simulink model "dynamics_old_3_12_24"  (R2023b)
settings: Solver=ode45  StartTime=0.0  StopTime=StopTime  FixedStep=.1  RelTol=1e-5
PreLoadFcn:
  | StopTime = 5000; gravity = true; k = 10; b = 100; ktr = 300; btr = 300; d0 = 125; l0 = 515.3882; mu = 398600000000000; mp = 1500; mp_inv = 0.00066667; mtr = 1.6667; mtr_inv = 0.6; NRao0 = [-504.021290494982;4.21156034226775e-10;6878000]; NRbo0 = [504.021290495824;4.21156034226775e-10;6878000]; NRfo0 = [4.21125171823769e-10;4.21125171823769e-10;6877495.9787095]; NRgo0 = [4.2118689662978e-10;4.2118689662978e-10;6878504.0212905]; NRdo0 = [4.21156034226775e-10;-124.968757810126;6878000]; NReo0 = [4.21156034226775e-10;124.968757810969;6878000]; NVao0 = [-7612.67977015526;-3.08624030053628e-16;-5.04021290495356]; NVbo0 = [-7612.67977015526;3.08624030053685e-16;5.04021290495449]; NVfo0 = [-7607.6395572503;2.85240796223787e-29;4.65833571642668e-13]; NVgo0 = [-7617.71998306021;2.85618751654332e-29;4.66450819702776e-13]; NVdo0 = [-7612.67977015526;2.85429773939059e-29;4.66142195672722e-13]; NVeo0 = [-7612.67977015526;2.85429773939059e-29;4.66142195672722e-13];
settings Model: Creator=cyrus  LastModifiedBy=cyrus

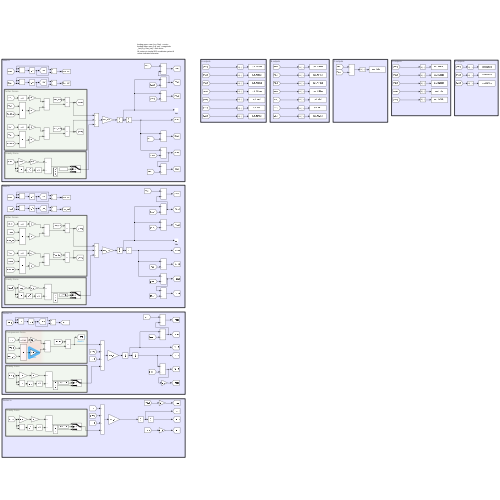
[thumbnail: Simulink's stored preview of the top-level diagram]
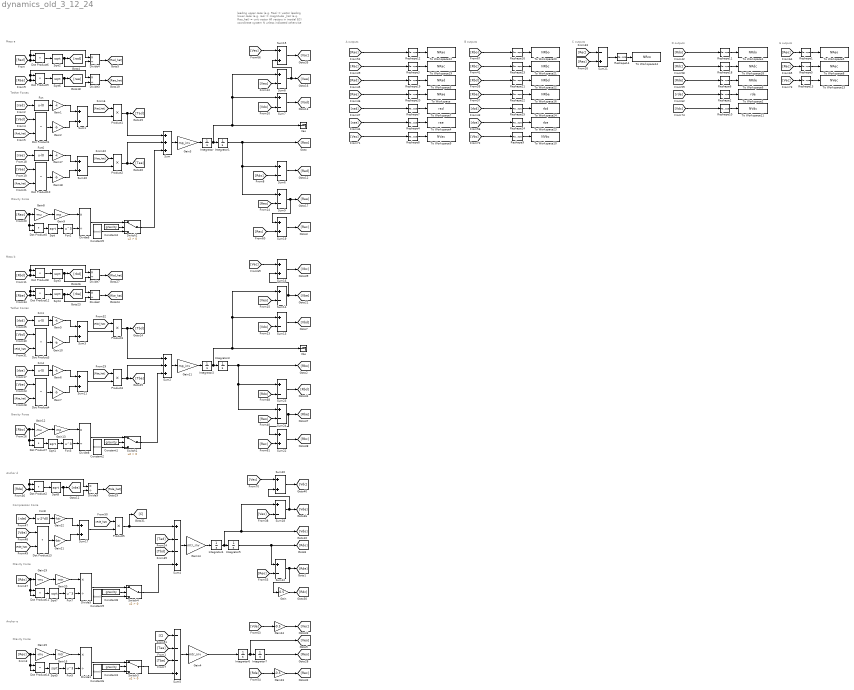
== system dynamics_old_3_12_24 ==
  note: A outputs
  note: Gravity Force
  note: Anchor d
  note: Tether Forces
  note: leading upper case (e.g. Rao) = vector
      | leading lower case (e.g. rao) = magnitude
      | _hat (e.g. Rao_hat) = unit vector
      | All vectors in inertial ECI coordinate system N unless indicated otherwise
  note: Mass a
  note: Gravity Force
  note: Gravity Force
  note: Tether Forces
  note: Mass b
  note: Gravity Force
  note: Anchor e
  note: Compression Force
  note: B outputs
  note: C outputs
  note: D outputs
  note: E outputs
  Constant{1,3..4,8} (4 alike) : Constant  Value=gravity
  Constant{2,5..6,9} (4 alike) : Constant  Value=[0;0;0]  VectorParams1D=off
  Divide{1..9} (9 alike) : Product  Inputs=*/
  Dot Product{1..14} (14 alike) : DotProduct  OutDataTypeStr=Inherit: Inherit via internal rule
  Fcn{,1,4,6} (4 alike) : Fcn  Expr=u-l0
  Fcn{2..3,5,7} (4 alike) : Fcn  Expr=u^3
  Fcn8 : Fcn  Expr=u-2*d0
  Gain : Gain  Gain=0.5
  Gain{1,5..6,17} (4 alike) : Gain  Gain=-k
  Gain{2,7,10,18} (4 alike) : Gain  Gain=-b
  Gain11 : Gain  Gain=mp_inv
  Gain{8,12,15,19} (4 alike) : Gain  Gain=-mu
  Gain13 : Gain  Gain=mp
  Gain14 : Gain  Gain=mtr_inv
  Gain16 : Gain  Gain=mtr
  Gain20 : Gain  Gain=mtr
  Gain21 : Gain  Gain=-btr
  Gain22 : Gain  Gain=-ktr
  Gain23 : Gain  Gain=-0.5
  Gain24 : Gain  Gain=-0.5
  Gain3 : Gain  Gain=mp_inv
  Gain4 : Gain  Gain=mtr_inv
  Gain9 : Gain  Gain=mp
  Integrator : Integrator  InitialCondition=NVao0
  Integrator1 : Integrator  InitialCondition=NRao0
  Integrator2 : Integrator  InitialCondition=NVbo0
  Integrator3 : Integrator  InitialCondition=NRbo0
  Integrator4 : Integrator  InitialCondition=NVdo0
  Integrator5 : Integrator  InitialCondition=NRdo0
  Integrator6 : Integrator  InitialCondition=NVeo0
  Integrator7 : Integrator  InitialCondition=NReo0
  Product{1..5} (5 alike) : Product
  Reshape{1..14,16,18..25} (23 alike) : Reshape
  Sqrt{,1..8} (9 alike) : Sqrt
  Sum : Sum  Inputs=+++
  Sum{1,3,10..11,15..17,19..20,22} (10 alike) : Sum
  Sum{6..9,12..14,18,23..24} (10 alike) : Sum  Inputs=+-
  Sum2 : Sum  Inputs=+++
  Sum21 : Sum  Inputs=-+
  Sum4 : Sum  Inputs=+--+
  Sum5 : Sum  Inputs=---+
  Switch{1..4} (4 alike) : Switch  Criteria=u2 > Threshold  SaturateOnIntegerOverflow=off  InputSameDT=off
  To Workspace : ToWorkspace  VariableName=NRae  SampleTime=-1
  To Workspace1 : ToWorkspace  VariableName=NRdo  SampleTime=-1
      settings: Save2DSignal=2-D array (concatenate along first dimension)
  To Workspace10 : ToWorkspace  VariableName=NVbc  SampleTime=-1
      settings: Save2DSignal=2-D array (concatenate along first dimension)
  To Workspace11 : ToWorkspace  VariableName=NVdc  SampleTime=-1
      settings: Save2DSignal=2-D array (concatenate along first dimension)
  To Workspace12 : ToWorkspace  VariableName=NRao  SampleTime=-1
      settings: Save2DSignal=2-D array (concatenate along first dimension)
  To Workspace13 : ToWorkspace  VariableName=NVec  SampleTime=-1
      settings: Save2DSignal=2-D array (concatenate along first dimension)
  To Workspace14 : ToWorkspace  VariableName=NRco  SampleTime=-1
      settings: Save2DSignal=2-D array (concatenate along first dimension)
  To Workspace16 : ToWorkspace  VariableName=NRbe  SampleTime=-1
  To Workspace18 : ToWorkspace  VariableName=NRdc  SampleTime=-1
      settings: Save2DSignal=2-D array (concatenate along first dimension)
  To Workspace19 : ToWorkspace  VariableName=NRac  SampleTime=-1
      settings: Save2DSignal=2-D array (concatenate along first dimension)
  To Workspace2 : ToWorkspace  VariableName=rde  SampleTime=-1
      settings: Save2DSignal=2-D array (concatenate along first dimension)
  To Workspace20 : ToWorkspace  VariableName=NRbo  SampleTime=-1
      settings: Save2DSignal=2-D array (concatenate along first dimension)
  To Workspace21 : ToWorkspace  VariableName=NRbc  SampleTime=-1
      settings: Save2DSignal=2-D array (concatenate along first dimension)
  To Workspace22 : ToWorkspace  VariableName=NRbd  SampleTime=-1
  To Workspace23 : ToWorkspace  VariableName=rbe  SampleTime=-1
      settings: Save2DSignal=2-D array (concatenate along first dimension)
  To Workspace24 : ToWorkspace  VariableName=rbd  SampleTime=-1
      settings: Save2DSignal=2-D array (concatenate along first dimension)
  To Workspace3 : ToWorkspace  VariableName=NRad  SampleTime=-1
  To Workspace4 : ToWorkspace  VariableName=rae  SampleTime=-1
      settings: Save2DSignal=2-D array (concatenate along first dimension)
  To Workspace5 : ToWorkspace  VariableName=NReo  SampleTime=-1
      settings: Save2DSignal=2-D array (concatenate along first dimension)
  To Workspace6 : ToWorkspace  VariableName=NRde  SampleTime=-1
      settings: Save2DSignal=2-D array (concatenate along first dimension)
  To Workspace7 : ToWorkspace  VariableName=rad  SampleTime=-1
      settings: Save2DSignal=2-D array (concatenate along first dimension)
  To Workspace8 : ToWorkspace  VariableName=NRec  SampleTime=-1
      settings: Save2DSignal=2-D array (concatenate along first dimension)
  To Workspace9 : ToWorkspace  VariableName=NVac  SampleTime=-1
      settings: Save2DSignal=2-D array (concatenate along first dimension)
  Vao : Terminator
  Vbo : Terminator
  wires:
  [Rad] -> Divide4/1, Dot Product6/1, Dot Product6/2
  Dot Product6/1 -> Sqrt2/1
  Sqrt2/1 -> Divide4/2, [rad]
  Divide4/1 -> [Rad_hat]
  [rad] -> Fcn/1
  Fcn/1 -> Gain1/1
  Gain1/1 -> Sum1/1
  [Vad] -> Dot Product1/1
  [Rad_hat] -> Dot Product1/2
  Dot Product1/1 -> Gain2/1
  Gain2/1 -> Sum1/2
  Sum1/1 -> Product1/2
  Sum/1 -> Gain3/1
  Gain3/1 -> Integrator/1
  Integrator/1 -> Integrator1/1, Vao/1, Sum7/1, Sum8/1
  Integrator1/1 -> [Rao], Sum6/1, Sum9/1
  [Rao] -> Dot Product5/2, Dot Product5/1, Gain8/1
  Gain8/1 -> Gain9/1
  Gain9/1 -> Divide6/1
  Fcn2/1 -> Divide6/2
  Sqrt/1 -> Fcn2/1
  Dot Product5/1 -> Sqrt/1
  Integrator4/1 -> Sum18/1, [Vdo], Integrator5/1
  Sum4/1 -> Gain14/1
  Integrator5/1 -> Sum12/1, [Rdo]
  Product1/1 -> Sum/1, [Tad]
  Constant4/1 -> Switch2/2
  Constant5/1 -> Switch2/3
  Divide6/1 -> Switch2/1
  Sum7/1 -> [Vad]
  [Vdo] -> Sum7/2
  [Veo] -> Sum8/2
  Sum8/1 -> Sum15/2, [Vae]
  Dot Product9/1 -> Sqrt6/1
  Sqrt6/1 -> Divide3/2, [rae]
  Divide3/1 -> [Rae_hat]
  [Rae] -> Divide3/1, Dot Product9/1, Dot Product9/2
  [Rad_hat] -> Product1/1
  Fcn6/1 -> Gain17/1
  [Vae] -> Dot Product10/1
  Product2/1 -> Sum/2, [Tae]
  Dot Product10/1 -> Gain18/1
  Gain17/1 -> Sum10/1
  Gain18/1 -> Sum10/2
  Sum10/1 -> Product2/2
  [rae] -> Fcn6/1
  [Rae_hat] -> Dot Product10/2
  [Rae_hat] -> Product2/1
  Switch2/1 -> Sum/3
  [Rdo] -> Dot Product11/2, Dot Product11/1, Gain19/1
  Divide5/1 -> Switch4/1
  Constant8/1 -> Switch4/2
  Constant9/1 -> Switch4/3
  Dot Product11/1 -> Sqrt7/1
  Gain19/1 -> Gain20/1
  Sqrt7/1 -> Fcn7/1
  Gain20/1 -> Divide5/1
  Fcn7/1 -> Divide5/2
  Switch1/1 -> Sum2/3
  [Rbe_hat] -> Dot Product4/2
  Sum11/1 -> Product4/2
  [rbe] -> Fcn4/1
  Product4/1 -> Sum2/2, [Tbe]
  Gain6/1 -> Sum11/1
  Gain7/1 -> Sum11/2
  Fcn4/1 -> Gain6/1
  [Vbe] -> Dot Product4/1
  Dot Product4/1 -> Gain7/1
  Sqrt4/1 -> Divide2/2, [rbe]
  [Rbe_hat] -> Product4/1
  [Vdo] -> Sum13/2
  Sum13/1 -> [Vbd]
  Sum14/1 -> Sum16/2, [Vbe]
  Dot Product12/1 -> Sqrt4/1
  [Veo] -> Sum14/2
  Fcn1/1 -> Gain5/1
  [Rbo] -> Dot Product7/2, Dot Product7/1, Gain12/1
  Divide2/1 -> [Rbe_hat]
  [Rbd_hat] -> Product3/1
  Divide8/1 -> Switch1/1
  Sum2/1 -> Gain11/1
  Constant1/1 -> Switch1/2
  Constant2/1 -> Switch1/3
  Sum3/1 -> Product3/2
  [Vbd] -> Dot Product3/1
  Fcn3/1 -> Divide8/2
  Dot Product8/1 -> Sqrt3/1
  Gain12/1 -> Gain13/1
  Sqrt1/1 -> Fcn3/1
  Gain13/1 -> Divide8/1
  Integrator3/1 -> Sum23/1, Sum24/1, [Rbo]
  Gain10/1 -> Sum3/2
  Dot Product3/1 -> Gain10/1
  Product3/1 -> Sum2/1, [Tbd]
  Gain5/1 -> Sum3/1
  [Rbe] -> Divide2/1, Dot Product12/1, Dot Product12/2
  [Rbd_hat] -> Dot Product3/2
  [rbd] -> Fcn1/1
  Sqrt3/1 -> Divide7/2, [rbd]
  Gain11/1 -> Integrator2/1
  Divide7/1 -> [Rbd_hat]
  Integrator2/1 -> Integrator3/1, Vbo/1, Sum13/1, Sum14/1
  Dot Product7/1 -> Sqrt1/1
  [Rbd] -> Divide7/1, Dot Product8/1, Dot Product8/2
  Constant6/1 -> Switch3/3
  Sum5/1 -> Gain4/1
  [Reo] -> Dot Product14/2, Dot Product14/1, Gain15/1
  Sqrt5/1 -> Fcn5/1
  Divide1/1 -> Switch3/1
  Constant3/1 -> Switch3/2
  Integrator7/1 -> [Reo]
  Integrator6/1 -> [Veo], Integrator7/1
  Gain15/1 -> Gain16/1
  Fcn5/1 -> Divide1/2
  Gain16/1 -> Divide1/1
  Dot Product14/1 -> Sqrt5/1
  Gain14/1 -> Integrator4/1
  Gain4/1 -> Integrator6/1
  Product5/1 -> Sum4/1, [C]
  [rde] -> Fcn8/1
  Dot Product13/1 -> Gain21/1
  Gain21/1 -> Sum17/2
  [Rde_hat] -> Product5/1
  [Rde_hat] -> Dot Product13/2
  Gain22/1 -> Sum17/1
  [Vde] -> Dot Product13/1
  Fcn8/1 -> Gain22/1
  Sum17/1 -> Product5/2
  Dot Product2/1 -> Sqrt8/1
  Divide9/1 -> [Rde_hat]
  Sqrt8/1 -> Divide9/2, [rde]
  [Rde] -> Divide9/1, Dot Product2/1, Dot Product2/2
  [Veo] -> Sum18/2
  Sum18/1 -> Sum20/2, [Vde]
  [Tbd] -> Sum4/3
  [Tad] -> Sum4/2
  Switch4/1 -> Sum4/4
  [Tbe] -> Sum5/3
  [Tae] -> Sum5/2
  Switch3/1 -> Sum5/4
  [C] -> Sum5/1
  Reshape12/1 -> To Workspace12/1
  [Rao] -> Reshape12/1
  Reshape19/1 -> To Workspace3/1
  Reshape20/1 -> To Workspace/1
  Reshape3/1 -> To Workspace19/1
  Reshape4/1 -> To Workspace4/1
  [rae] -> Reshape4/1
  [rad] -> Reshape7/1
  Reshape7/1 -> To Workspace7/1
  Reshape23/1 -> To Workspace21/1
  Reshape21/1 -> To Workspace22/1
  Reshape25/1 -> To Workspace24/1
  Reshape24/1 -> To Workspace23/1
  [rbe] -> Reshape24/1
  [rbd] -> Reshape25/1
  [Rbo] -> Reshape16/1
  Reshape22/1 -> To Workspace16/1
  Reshape16/1 -> To Workspace20/1
  Sum21/1 -> Reshape14/1
  [Rec] -> Sum21/1
  [Reo] -> Sum21/2
  Reshape14/1 -> To Workspace14/1
  [Rdo] -> Sum6/2
  Sum6/1 -> [Rad]
  [Reo] -> Sum9/2
  Sum9/1 -> Sum19/1, [Rae]
  [Rad] -> Reshape19/1
  [Rae] -> Reshape20/1
  [Rec] -> Sum19/2
  Sum19/1 -> [Rac]
  [Rac] -> Reshape3/1
  [Reo] -> Sum24/2
  [Rdo] -> Sum23/2
  Sum23/1 -> [Rbd]
  Sum24/1 -> Sum22/1, [Rbe]
  Sum22/1 -> [Rbc]
  [Rec] -> Sum22/2
  [Rbc] -> Reshape23/1
  [Rbd] -> Reshape21/1
  [Rbe] -> Reshape22/1
  Sum12/1 -> Gain/1, [Rde]
  [Reo] -> Sum12/2
  Gain/1 -> [Rdc]
  [Rdo] -> Reshape11/1
  Reshape11/1 -> To Workspace1/1
  Reshape6/1 -> To Workspace6/1
  Reshape2/1 -> To Workspace2/1
  Reshape18/1 -> To Workspace18/1
  [Rdc] -> Reshape18/1
  [Rde] -> Reshape6/1
  [rde] -> Reshape2/1
  [Reo] -> Reshape1/1
  Reshape1/1 -> To Workspace5/1
  [Rec] -> Reshape5/1
  Reshape5/1 -> To Workspace8/1
  Gain23/1 -> [Rec]
  [Rde] -> Gain23/1
  [Vde] -> Gain24/1
  Gain24/1 -> [Vec]
  Sum15/1 -> [Vac]
  [Vec] -> Sum15/1
  Sum16/1 -> [Vbc]
  [Vec] -> Sum16/1
  [Vec] -> Sum20/1
  Sum20/1 -> [Vdc]
  [Vac] -> Reshape8/1
  Reshape8/1 -> To Workspace9/1
  Reshape9/1 -> To Workspace10/1
  [Vbc] -> Reshape9/1
  Reshape10/1 -> To Workspace11/1
  [Vdc] -> Reshape10/1
  Reshape13/1 -> To Workspace13/1
  [Vec] -> Reshape13/1
